simulink model "model_feedback"  (R2023b)
settings: Solver=VariableStepAuto  StartTime=0.0  StopTime=5  RelTol=1e-3
libraries: simulink_extras x5, spspowerguiLib x1
settings Model: Creator=dimia  LastModifiedBy=dimia

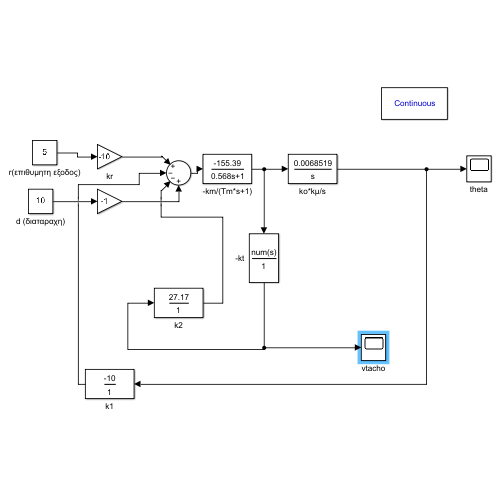
[thumbnail: Simulink's stored preview of the top-level diagram]
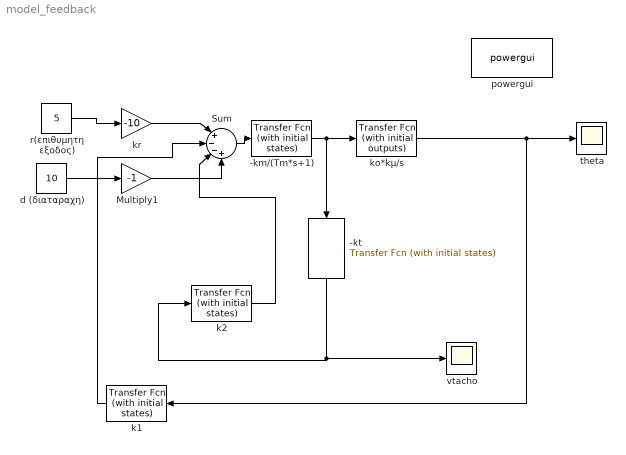
== system model_feedback ==
  -km/(Tm*s+1) : simulink_extras/Additional Linear/Transfer Fcn (with initial states)  N=[-155.39]  D="[0.568  1]"  X0=0
  -kt : simulink_extras/Additional Linear/Transfer Fcn (with initial states)  N=-9.2667*10^(-4)  D=[1]  X0=0
  Multiply1 : Gain  Gain=-1
  Sum : Sum  Inputs=|+--+
  d (διαταραχη) : Constant  Value=10
  k1 : simulink_extras/Additional Linear/Transfer Fcn (with initial states)  N=[-10]  D=[1]  X0=0
  k2 : simulink_extras/Additional Linear/Transfer Fcn (with initial states)  N=27.17  D=[1]  X0=0
  ko*kμ/s : simulink_extras/Additional Linear/Transfer Fcn (with initial outputs)  N=[(1/36)*0.24667]  D="[1  0]"  Y0=2  U0=0
  kr : Gain  Gain=-10
  powergui : spspowerguiLib/powergui  Priority=1  SimulationMode=Continuous  SampleTime=50e-6  frequency=60  Iterations=50  frequencyindice=60  Pbase=100e6  ErrMax=1e-4  UnitsV=kV  UnitsW=MW  buscounter=0  FunctionMessages=off  echomessages=off  EnableUseOfTLC=off  CurrentSourceSwitches=off  DisableSnubberDevices=off  DisableRonSwitches=off  DisableVfSwitches=off  DisplayEquations=off  AutomaticDiscreteSolvers=off  SolverType=Tustin/Backward Euler (TBE)  Interpol=off  ExternalGateDelay=off  methode=off  Ts=100  x0status=blocks  SPID=on  SwTol=0  HookPort=off  NonlinearTolerance=1e-4  nMaxIteration=100  ContinueOnMaxIteration=off  RestoreLinks=warning  ResistiveCurrentMeasurement=off  Frange=[0:2:500]  Ylog=off  Xlog=on  ShowGrid=off  save=off  variable=ZData  structure=0  ZoomFFT=off  StartTime=0.0  cycles=1  DisplayStyle=1  fundamental=60  FreqAxis=off  MaxFrequency=1000  frequencyindicesteady=1  RmsSteady=1  display=off
  r(επιθυμητη εξοδος) : Constant  Value=5  VectorParams1D=off
  theta : Scope
  vtacho : Scope
  wires:
  -km/(Tm*s+1)/1 -> ko*kμ/s/1, -kt/1
  kr/1 -> Sum/1
  -kt/1 -> k2/1, vtacho/1
  ko*kμ/s/1 -> k1/1, theta/1
  Sum/1 -> -km/(Tm*s+1)/1
  k2/1 -> Sum/3
  k1/1 -> Sum/2
  d (διαταραχη)/1 -> Multiply1/1
  r(επιθυμητη εξοδος)/1 -> kr/1
  Multiply1/1 -> Sum/4
